simulink subsystem "ElectricalThermalSystem"  (R2025b)
settings: Solver=VariableStepAuto  StartTime=0.0  StopTime=10.0  RelTol=1e-3
undefined symbols (not defined in the file): EnvAirTemp, PlantThrEstCmpPwr, PlntThrAirBpt, PlntThrAirCond, PlntThrAirCp, PlntThrAirCpBpt, PlntThrAirPrand, PlntThrAirRho, PlntThrAirVisc, PlntThrBattDCFlwRatio, PlntThrBattJacLen, PlntThrChArea, PlntThrChDia, PlntThrCoolCond, PlntThrCoolCp, PlntThrCoolCpBpt, PlntThrCoolPrand, PlntThrCoolRho, PlntThrCoolVisc, PlntThrDCJacLen, PlntThrEMJacLen, PlntThrEstCOPLut, PlntThrEstDTLut, PlntThrHeaterMaxPwr, PlntThrPmpDisp, PlntThrPmpHeadP, PlntThrPmpMaxSpd, PlntThrPmpMechEff, PlntThrPmpVolEff, PlntThrRadAirArea, PlntThrRadAirDh, PlntThrRadFanAreaFlw, PlntThrRadFlwCoef, PlntThrRadGapHeight, PlntThrRadLength, PlntThrRadNTubes, PlntThrRadTubeDh, PlntThrRadTubeHeight, PlntThrRadWidth
libraries: autolibutils x62
(part 4 of 4)

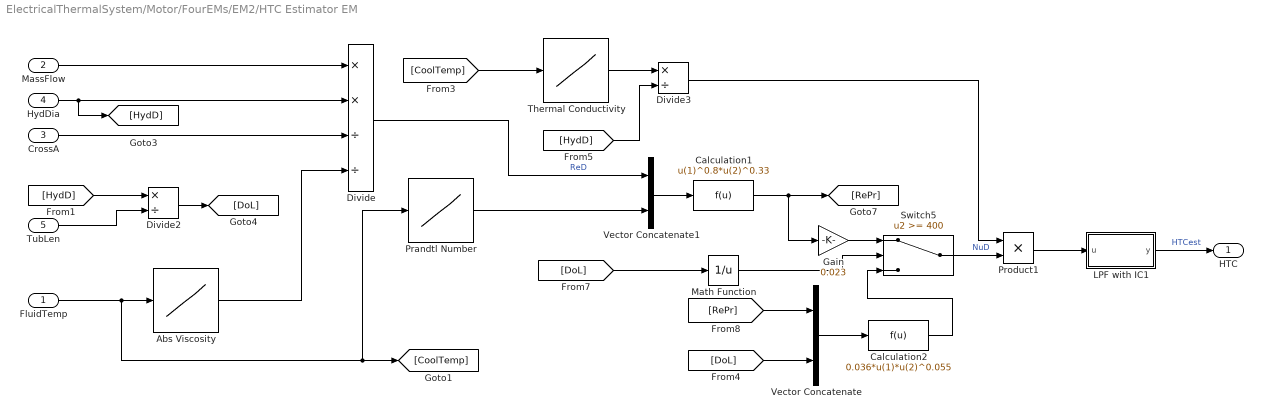
== system ElectricalThermalSystem/Motor/FourEMs/EM2/HTC Estimator EM ==
  FluidTemp : Inport
  MassFlow : Inport  Port=2
  CrossA : Inport  Port=3  OutMin=eps
  HydDia : Inport  Port=4
  TubLen : Inport  Port=5
  Abs Viscosity : Lookup_n-D  NumberOfTableDimensions=1  BreakpointsForDimension1=PlntThrCoolCpBpt  Table=PlntThrCoolVisc  ExtrapMethod=Clip  UseLastTableValue=on  InternalRulePriority=Speed  RndMeth=Simplest
  Calculation1 : Fcn  Expr=u(1)^0.8*u(2)^0.33
  Calculation2 : Fcn  Expr=0.036*u(1)*u(2)^0.055
  Divide : Product  Inputs=**//
  Divide2 : Product  Inputs=*/
  Divide3 : Product  Inputs=*/
  Gain : Gain  Gain=0.023
  LPF with IC1 : Subsystem  mask{wc=10, InitCond=10, dataType=off}
      mask prompts: wc "Cutoff frequency, wc [rad/s]"; InitCond "Initial condition, InitCond [same as u]"; dataType "Enforce same input data type"
      mask TypeOptions wc: Cont LPF IC/wc
      mask TypeOptions InitCond: Initial Condition/Value
      mask TypeOptions dataType: Cont LPF IC/dataType
  Math Function : Math  Operator=reciprocal
  Prandtl Number : Lookup_n-D  NumberOfTableDimensions=1  BreakpointsForDimension1=PlntThrCoolCpBpt  Table=PlntThrCoolPrand  ExtrapMethod=Clip  UseLastTableValue=on  InternalRulePriority=Speed  RndMeth=Simplest
  Product1 : Product
  Switch5 : Switch  Threshold=400  SaturateOnIntegerOverflow=off  InputSameDT=off
  Thermal Conductivity : Lookup_n-D  NumberOfTableDimensions=1  BreakpointsForDimension1=PlntThrCoolCpBpt  Table=PlntThrCoolCond  ExtrapMethod=Clip  UseLastTableValue=on  InternalRulePriority=Speed  RndMeth=Simplest
  Vector Concatenate : Concatenate
  Vector Concatenate1 : Concatenate
  HTC : Outport
  wires:
  LPF with IC1/1(y) -> HTC/1  "HTCest"
  FluidTemp/1 -> Prandtl Number/1, [CoolTemp], Abs Viscosity/1
  [CoolTemp] -> Thermal Conductivity/1
  MassFlow/1 -> Divide/1
  HydDia/1 -> [HydD], Divide/2
  CrossA/1 -> Divide/3
  [HydD] -> Divide2/1
  TubLen/1 -> Divide2/2
  Divide2/1 -> [DoL]
  Abs Viscosity/1 -> Divide/4
  Divide/1 -> Vector Concatenate1/1  "ReD"
  Prandtl Number/1 -> Vector Concatenate1/2
  Vector Concatenate1/1 -> Calculation1/1
  [DoL] -> Math Function/1
  Math Function/1 -> Switch5/2
  Thermal Conductivity/1 -> Divide3/1
  [HydD] -> Divide3/2
  Divide3/1 -> Product1/1
  Gain/1 -> Switch5/1
  Calculation1/1 -> [RePr], Gain/1
  [RePr] -> Vector Concatenate/1
  [DoL] -> Vector Concatenate/2
  Vector Concatenate/1 -> Calculation2/1
  Calculation2/1 -> Switch5/3
  Switch5/1 -> Product1/2  "NuD"
  Product1/1 -> LPF with IC1/1(u)

== system ElectricalThermalSystem/Motor/FourEMs/EM2/Temperature and Heat Flow ==
  HTC : Inport
  CoolTempIn : Inport  Port=2
  EMTemp : Inport  Port=3
  CoolMflw : Inport  Port=4
  JacArea : Inport  Port=5
  Divide2 : Product  Inputs=*/
  Gain4 : Gain  Gain=0.5
  LPF with IC1 : Subsystem  mask{wc=10, InitCond=EnvAirTemp, dataType=off}
      mask prompts: wc "Cutoff frequency, wc [rad/s]"; InitCond "Initial condition, InitCond [same as u]"; dataType "Enforce same input data type"
      mask TypeOptions wc: Cont LPF IC/wc
      mask TypeOptions InitCond: Initial Condition/Value
      mask TypeOptions dataType: Cont LPF IC/dataType
  Minus3 : Sum
  Minus4 : Sum
  Product1 : Product  Inputs=3
  Product2 : Product
  Selector : Selector  InputPortWidth=PlntEMNum  IndexOptions=Index vector (dialog)  Indices=2  OutputSizes=1
  Specific Heat 2 : Lookup_n-D  NumberOfTableDimensions=1  BreakpointsForDimension1=PlntThrCoolCpBpt  Table=PlntThrCoolCp  ExtrapMethod=Clip  UseLastTableValue=on  InternalRulePriority=Speed  RndMeth=Simplest
  Subtract : Sum  Inputs=+-
  div0protect - abs poly4 : autolibutils/div0protect - abs poly  thresh=.001  aMode=1
  BulkCoolTemp : Outport
  Qem : Outport  Port=2
  CoolTempOut : Outport  Port=3
  wires:
  LPF with IC1/1(y) -> BulkCoolTemp/1, [BulkCoolTemp]
  EMTemp/1 -> Selector/1
  HTC/1 -> Product1/1
  Product2/1 -> div0protect - abs poly4/1
  Minus4/1 -> Gain4/1
  Gain4/1 -> LPF with IC1/1(u)
  Minus3/1 -> Minus4/2, CoolTempOut/1
  Product1/1 -> Divide2/1, Qem/1  "Qem"
  JacArea/1 -> Product1/2
  div0protect - abs poly4/1 -> Divide2/2
  Specific Heat 2/1 -> Product2/2
  [BulkCoolTemp] -> Specific Heat 2/1, Subtract/2
  Subtract/1 -> Product1/3
  Selector/1 -> Subtract/1
  Divide2/1 -> Minus3/2
  CoolMflw/1 -> Product2/1
  CoolTempIn/1 -> Minus4/1, Minus3/1

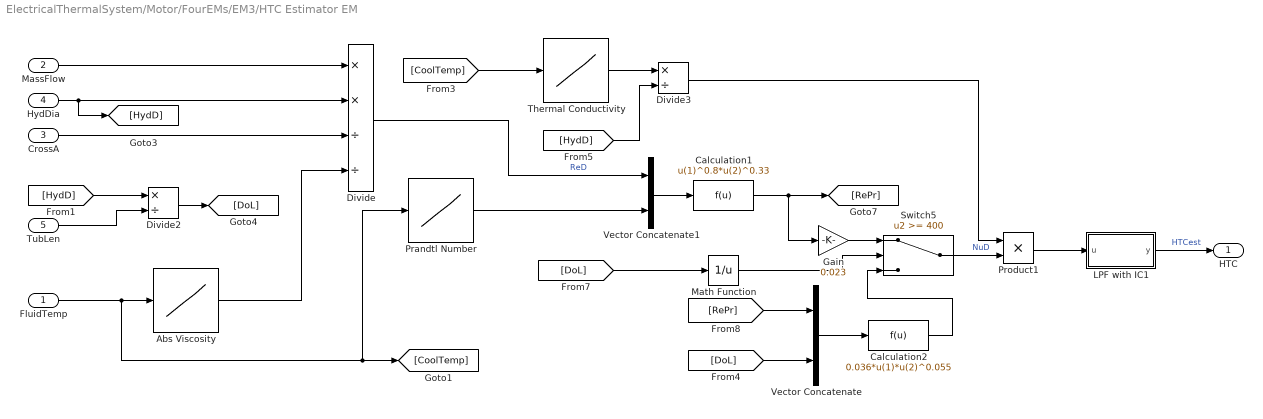
== system ElectricalThermalSystem/Motor/FourEMs/EM3/HTC Estimator EM ==
  FluidTemp : Inport
  MassFlow : Inport  Port=2
  CrossA : Inport  Port=3  OutMin=eps
  HydDia : Inport  Port=4
  TubLen : Inport  Port=5
  Abs Viscosity : Lookup_n-D  NumberOfTableDimensions=1  BreakpointsForDimension1=PlntThrCoolCpBpt  Table=PlntThrCoolVisc  ExtrapMethod=Clip  UseLastTableValue=on  InternalRulePriority=Speed  RndMeth=Simplest
  Calculation1 : Fcn  Expr=u(1)^0.8*u(2)^0.33
  Calculation2 : Fcn  Expr=0.036*u(1)*u(2)^0.055
  Divide : Product  Inputs=**//
  Divide2 : Product  Inputs=*/
  Divide3 : Product  Inputs=*/
  Gain : Gain  Gain=0.023
  LPF with IC1 : Subsystem  mask{wc=10, InitCond=10, dataType=off}
      mask prompts: wc "Cutoff frequency, wc [rad/s]"; InitCond "Initial condition, InitCond [same as u]"; dataType "Enforce same input data type"
      mask TypeOptions wc: Cont LPF IC/wc
      mask TypeOptions InitCond: Initial Condition/Value
      mask TypeOptions dataType: Cont LPF IC/dataType
  Math Function : Math  Operator=reciprocal
  Prandtl Number : Lookup_n-D  NumberOfTableDimensions=1  BreakpointsForDimension1=PlntThrCoolCpBpt  Table=PlntThrCoolPrand  ExtrapMethod=Clip  UseLastTableValue=on  InternalRulePriority=Speed  RndMeth=Simplest
  Product1 : Product
  Switch5 : Switch  Threshold=400  SaturateOnIntegerOverflow=off  InputSameDT=off
  Thermal Conductivity : Lookup_n-D  NumberOfTableDimensions=1  BreakpointsForDimension1=PlntThrCoolCpBpt  Table=PlntThrCoolCond  ExtrapMethod=Clip  UseLastTableValue=on  InternalRulePriority=Speed  RndMeth=Simplest
  Vector Concatenate : Concatenate
  Vector Concatenate1 : Concatenate
  HTC : Outport
  wires:
  LPF with IC1/1(y) -> HTC/1  "HTCest"
  FluidTemp/1 -> Prandtl Number/1, [CoolTemp], Abs Viscosity/1
  [CoolTemp] -> Thermal Conductivity/1
  MassFlow/1 -> Divide/1
  HydDia/1 -> [HydD], Divide/2
  CrossA/1 -> Divide/3
  [HydD] -> Divide2/1
  TubLen/1 -> Divide2/2
  Divide2/1 -> [DoL]
  Abs Viscosity/1 -> Divide/4
  Divide/1 -> Vector Concatenate1/1  "ReD"
  Prandtl Number/1 -> Vector Concatenate1/2
  Vector Concatenate1/1 -> Calculation1/1
  [DoL] -> Math Function/1
  Math Function/1 -> Switch5/2
  Thermal Conductivity/1 -> Divide3/1
  [HydD] -> Divide3/2
  Divide3/1 -> Product1/1
  Gain/1 -> Switch5/1
  Calculation1/1 -> [RePr], Gain/1
  [RePr] -> Vector Concatenate/1
  [DoL] -> Vector Concatenate/2
  Vector Concatenate/1 -> Calculation2/1
  Calculation2/1 -> Switch5/3
  Switch5/1 -> Product1/2  "NuD"
  Product1/1 -> LPF with IC1/1(u)

== system ElectricalThermalSystem/Motor/FourEMs/EM3/Temperature and Heat Flow ==
  HTC : Inport
  CoolTempIn : Inport  Port=2
  EMTemp : Inport  Port=3
  CoolMflw : Inport  Port=4
  JacArea : Inport  Port=5
  Divide2 : Product  Inputs=*/
  Gain4 : Gain  Gain=0.5
  LPF with IC1 : Subsystem  mask{wc=10, InitCond=EnvAirTemp, dataType=off}
      mask prompts: wc "Cutoff frequency, wc [rad/s]"; InitCond "Initial condition, InitCond [same as u]"; dataType "Enforce same input data type"
      mask TypeOptions wc: Cont LPF IC/wc
      mask TypeOptions InitCond: Initial Condition/Value
      mask TypeOptions dataType: Cont LPF IC/dataType
  Minus3 : Sum
  Minus4 : Sum
  Product1 : Product  Inputs=3
  Product2 : Product
  Selector : Selector  InputPortWidth=PlntEMNum  IndexOptions=Index vector (dialog)  Indices=3  OutputSizes=1
  Specific Heat 2 : Lookup_n-D  NumberOfTableDimensions=1  BreakpointsForDimension1=PlntThrCoolCpBpt  Table=PlntThrCoolCp  ExtrapMethod=Clip  UseLastTableValue=on  InternalRulePriority=Speed  RndMeth=Simplest
  Subtract : Sum  Inputs=+-
  div0protect - abs poly4 : autolibutils/div0protect - abs poly  thresh=.001  aMode=1
  BulkCoolTemp : Outport
  Qem : Outport  Port=2
  CoolTempOut : Outport  Port=3
  wires:
  LPF with IC1/1(y) -> BulkCoolTemp/1, [BulkCoolTemp]
  EMTemp/1 -> Selector/1
  HTC/1 -> Product1/1
  Product2/1 -> div0protect - abs poly4/1
  Minus4/1 -> Gain4/1
  Gain4/1 -> LPF with IC1/1(u)
  Minus3/1 -> Minus4/2, CoolTempOut/1
  Product1/1 -> Divide2/1, Qem/1  "Qem"
  JacArea/1 -> Product1/2
  div0protect - abs poly4/1 -> Divide2/2
  Specific Heat 2/1 -> Product2/2
  [BulkCoolTemp] -> Specific Heat 2/1, Subtract/2
  Subtract/1 -> Product1/3
  Selector/1 -> Subtract/1
  Divide2/1 -> Minus3/2
  CoolMflw/1 -> Product2/1
  CoolTempIn/1 -> Minus4/1, Minus3/1

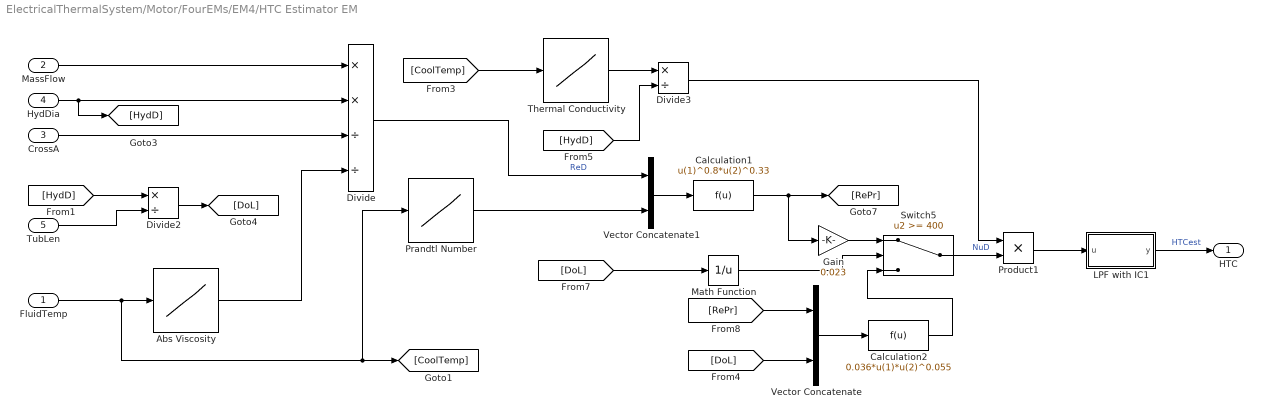
== system ElectricalThermalSystem/Motor/FourEMs/EM4/HTC Estimator EM ==
  FluidTemp : Inport
  MassFlow : Inport  Port=2
  CrossA : Inport  Port=3  OutMin=eps
  HydDia : Inport  Port=4
  TubLen : Inport  Port=5
  Abs Viscosity : Lookup_n-D  NumberOfTableDimensions=1  BreakpointsForDimension1=PlntThrCoolCpBpt  Table=PlntThrCoolVisc  ExtrapMethod=Clip  UseLastTableValue=on  InternalRulePriority=Speed  RndMeth=Simplest
  Calculation1 : Fcn  Expr=u(1)^0.8*u(2)^0.33
  Calculation2 : Fcn  Expr=0.036*u(1)*u(2)^0.055
  Divide : Product  Inputs=**//
  Divide2 : Product  Inputs=*/
  Divide3 : Product  Inputs=*/
  Gain : Gain  Gain=0.023
  LPF with IC1 : Subsystem  mask{wc=10, InitCond=10, dataType=off}
      mask prompts: wc "Cutoff frequency, wc [rad/s]"; InitCond "Initial condition, InitCond [same as u]"; dataType "Enforce same input data type"
      mask TypeOptions wc: Cont LPF IC/wc
      mask TypeOptions InitCond: Initial Condition/Value
      mask TypeOptions dataType: Cont LPF IC/dataType
  Math Function : Math  Operator=reciprocal
  Prandtl Number : Lookup_n-D  NumberOfTableDimensions=1  BreakpointsForDimension1=PlntThrCoolCpBpt  Table=PlntThrCoolPrand  ExtrapMethod=Clip  UseLastTableValue=on  InternalRulePriority=Speed  RndMeth=Simplest
  Product1 : Product
  Switch5 : Switch  Threshold=400  SaturateOnIntegerOverflow=off  InputSameDT=off
  Thermal Conductivity : Lookup_n-D  NumberOfTableDimensions=1  BreakpointsForDimension1=PlntThrCoolCpBpt  Table=PlntThrCoolCond  ExtrapMethod=Clip  UseLastTableValue=on  InternalRulePriority=Speed  RndMeth=Simplest
  Vector Concatenate : Concatenate
  Vector Concatenate1 : Concatenate
  HTC : Outport
  wires:
  LPF with IC1/1(y) -> HTC/1  "HTCest"
  FluidTemp/1 -> Prandtl Number/1, [CoolTemp], Abs Viscosity/1
  [CoolTemp] -> Thermal Conductivity/1
  MassFlow/1 -> Divide/1
  HydDia/1 -> [HydD], Divide/2
  CrossA/1 -> Divide/3
  [HydD] -> Divide2/1
  TubLen/1 -> Divide2/2
  Divide2/1 -> [DoL]
  Abs Viscosity/1 -> Divide/4
  Divide/1 -> Vector Concatenate1/1  "ReD"
  Prandtl Number/1 -> Vector Concatenate1/2
  Vector Concatenate1/1 -> Calculation1/1
  [DoL] -> Math Function/1
  Math Function/1 -> Switch5/2
  Thermal Conductivity/1 -> Divide3/1
  [HydD] -> Divide3/2
  Divide3/1 -> Product1/1
  Gain/1 -> Switch5/1
  Calculation1/1 -> [RePr], Gain/1
  [RePr] -> Vector Concatenate/1
  [DoL] -> Vector Concatenate/2
  Vector Concatenate/1 -> Calculation2/1
  Calculation2/1 -> Switch5/3
  Switch5/1 -> Product1/2  "NuD"
  Product1/1 -> LPF with IC1/1(u)

== system ElectricalThermalSystem/Motor/FourEMs/EM4/Temperature and Heat Flow ==
  HTC : Inport
  CoolTempIn : Inport  Port=2
  EMTemp : Inport  Port=3
  CoolMflw : Inport  Port=4
  JacArea : Inport  Port=5
  Divide2 : Product  Inputs=*/
  Gain4 : Gain  Gain=0.5
  LPF with IC1 : Subsystem  mask{wc=10, InitCond=EnvAirTemp, dataType=off}
      mask prompts: wc "Cutoff frequency, wc [rad/s]"; InitCond "Initial condition, InitCond [same as u]"; dataType "Enforce same input data type"
      mask TypeOptions wc: Cont LPF IC/wc
      mask TypeOptions InitCond: Initial Condition/Value
      mask TypeOptions dataType: Cont LPF IC/dataType
  Minus3 : Sum
  Minus4 : Sum
  Product1 : Product  Inputs=3
  Product2 : Product
  Selector : Selector  InputPortWidth=PlntEMNum  IndexOptions=Index vector (dialog)  Indices=4  OutputSizes=1
  Specific Heat 2 : Lookup_n-D  NumberOfTableDimensions=1  BreakpointsForDimension1=PlntThrCoolCpBpt  Table=PlntThrCoolCp  ExtrapMethod=Clip  UseLastTableValue=on  InternalRulePriority=Speed  RndMeth=Simplest
  Subtract : Sum  Inputs=+-
  div0protect - abs poly4 : autolibutils/div0protect - abs poly  thresh=.001  aMode=1
  BulkCoolTemp : Outport
  Qem : Outport  Port=2
  CoolTempOut : Outport  Port=3
  wires:
  LPF with IC1/1(y) -> BulkCoolTemp/1, [BulkCoolTemp]
  EMTemp/1 -> Selector/1
  HTC/1 -> Product1/1
  Product2/1 -> div0protect - abs poly4/1
  Minus4/1 -> Gain4/1
  Gain4/1 -> LPF with IC1/1(u)
  Minus3/1 -> Minus4/2, CoolTempOut/1
  Product1/1 -> Divide2/1, Qem/1  "Qem"
  JacArea/1 -> Product1/2
  div0protect - abs poly4/1 -> Divide2/2
  Specific Heat 2/1 -> Product2/2
  [BulkCoolTemp] -> Specific Heat 2/1, Subtract/2
  Subtract/1 -> Product1/3
  Selector/1 -> Subtract/1
  Divide2/1 -> Minus3/2
  CoolMflw/1 -> Product2/1
  CoolTempIn/1 -> Minus4/1, Minus3/1

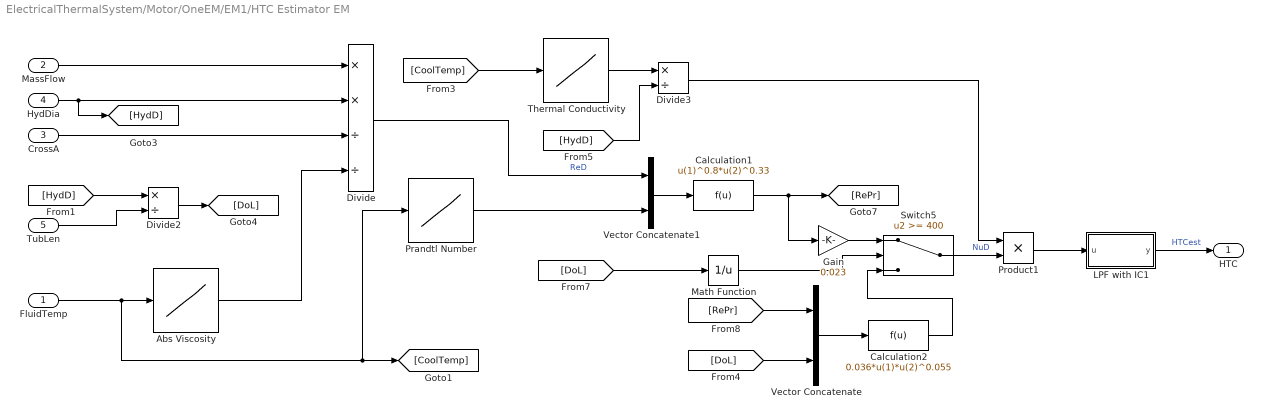
== system ElectricalThermalSystem/Motor/OneEM/EM1/HTC Estimator EM ==
  FluidTemp : Inport
  MassFlow : Inport  Port=2
  CrossA : Inport  Port=3  OutMin=eps
  HydDia : Inport  Port=4
  TubLen : Inport  Port=5
  Abs Viscosity : Lookup_n-D  NumberOfTableDimensions=1  BreakpointsForDimension1=PlntThrCoolCpBpt  Table=PlntThrCoolVisc  ExtrapMethod=Clip  UseLastTableValue=on  InternalRulePriority=Speed  RndMeth=Simplest
  Calculation1 : Fcn  Expr=u(1)^0.8*u(2)^0.33
  Calculation2 : Fcn  Expr=0.036*u(1)*u(2)^0.055
  Divide : Product  Inputs=**//
  Divide2 : Product  Inputs=*/
  Divide3 : Product  Inputs=*/
  Gain : Gain  Gain=0.023
  LPF with IC1 : Subsystem  mask{wc=10, InitCond=10, dataType=off}
      mask prompts: wc "Cutoff frequency, wc [rad/s]"; InitCond "Initial condition, InitCond [same as u]"; dataType "Enforce same input data type"
      mask TypeOptions wc: Cont LPF IC/wc
      mask TypeOptions InitCond: Initial Condition/Value
      mask TypeOptions dataType: Cont LPF IC/dataType
  Math Function : Math  Operator=reciprocal
  Prandtl Number : Lookup_n-D  NumberOfTableDimensions=1  BreakpointsForDimension1=PlntThrCoolCpBpt  Table=PlntThrCoolPrand  ExtrapMethod=Clip  UseLastTableValue=on  InternalRulePriority=Speed  RndMeth=Simplest
  Product1 : Product
  Switch5 : Switch  Threshold=400  SaturateOnIntegerOverflow=off  InputSameDT=off
  Thermal Conductivity : Lookup_n-D  NumberOfTableDimensions=1  BreakpointsForDimension1=PlntThrCoolCpBpt  Table=PlntThrCoolCond  ExtrapMethod=Clip  UseLastTableValue=on  InternalRulePriority=Speed  RndMeth=Simplest
  Vector Concatenate : Concatenate
  Vector Concatenate1 : Concatenate
  HTC : Outport
  wires:
  LPF with IC1/1(y) -> HTC/1  "HTCest"
  FluidTemp/1 -> Prandtl Number/1, [CoolTemp], Abs Viscosity/1
  [CoolTemp] -> Thermal Conductivity/1
  MassFlow/1 -> Divide/1
  HydDia/1 -> [HydD], Divide/2
  CrossA/1 -> Divide/3
  [HydD] -> Divide2/1
  TubLen/1 -> Divide2/2
  Divide2/1 -> [DoL]
  Abs Viscosity/1 -> Divide/4
  Divide/1 -> Vector Concatenate1/1  "ReD"
  Prandtl Number/1 -> Vector Concatenate1/2
  Vector Concatenate1/1 -> Calculation1/1
  [DoL] -> Math Function/1
  Math Function/1 -> Switch5/2
  Thermal Conductivity/1 -> Divide3/1
  [HydD] -> Divide3/2
  Divide3/1 -> Product1/1
  Gain/1 -> Switch5/1
  Calculation1/1 -> [RePr], Gain/1
  [RePr] -> Vector Concatenate/1
  [DoL] -> Vector Concatenate/2
  Vector Concatenate/1 -> Calculation2/1
  Calculation2/1 -> Switch5/3
  Switch5/1 -> Product1/2  "NuD"
  Product1/1 -> LPF with IC1/1(u)

== system ElectricalThermalSystem/Motor/OneEM/EM1/Temperature and Heat Flow ==
  HTC : Inport
  CoolTempIn : Inport  Port=2
  EMTemp : Inport  Port=3
  CoolMflw : Inport  Port=4
  JacArea : Inport  Port=5
  Divide2 : Product  Inputs=*/
  Gain4 : Gain  Gain=0.5
  LPF with IC1 : Subsystem  mask{wc=10, InitCond=EnvAirTemp, dataType=off}
      mask prompts: wc "Cutoff frequency, wc [rad/s]"; InitCond "Initial condition, InitCond [same as u]"; dataType "Enforce same input data type"
      mask TypeOptions wc: Cont LPF IC/wc
      mask TypeOptions InitCond: Initial Condition/Value
      mask TypeOptions dataType: Cont LPF IC/dataType
  Minus3 : Sum
  Minus4 : Sum
  Product1 : Product  Inputs=3
  Product2 : Product
  Selector : Selector  InputPortWidth=PlntEMNum  IndexOptions=Index vector (dialog)  Indices=1  OutputSizes=1
  Specific Heat 2 : Lookup_n-D  NumberOfTableDimensions=1  BreakpointsForDimension1=PlntThrCoolCpBpt  Table=PlntThrCoolCp  ExtrapMethod=Clip  UseLastTableValue=on  InternalRulePriority=Speed  RndMeth=Simplest
  Subtract : Sum  Inputs=+-
  div0protect - abs poly4 : autolibutils/div0protect - abs poly  thresh=.001  aMode=1
  BulkCoolTemp : Outport
  Qem : Outport  Port=2
  CoolTempOut : Outport  Port=3
  wires:
  LPF with IC1/1(y) -> BulkCoolTemp/1, [BulkCoolTemp]
  EMTemp/1 -> Selector/1
  HTC/1 -> Product1/1
  Product2/1 -> div0protect - abs poly4/1
  Minus4/1 -> Gain4/1
  Gain4/1 -> LPF with IC1/1(u)
  Minus3/1 -> Minus4/2, CoolTempOut/1
  Product1/1 -> Divide2/1, Qem/1  "Qem"
  JacArea/1 -> Product1/2
  div0protect - abs poly4/1 -> Divide2/2
  Specific Heat 2/1 -> Product2/2
  [BulkCoolTemp] -> Specific Heat 2/1, Subtract/2
  Subtract/1 -> Product1/3
  Selector/1 -> Subtract/1
  Divide2/1 -> Minus3/2
  CoolMflw/1 -> Product2/1
  CoolTempIn/1 -> Minus4/1, Minus3/1

== system ElectricalThermalSystem/Motor/ThreeEMs/EM1/HTC Estimator EM ==
  FluidTemp : Inport
  MassFlow : Inport  Port=2
  CrossA : Inport  Port=3  OutMin=eps
  HydDia : Inport  Port=4
  TubLen : Inport  Port=5
  Abs Viscosity : Lookup_n-D  NumberOfTableDimensions=1  BreakpointsForDimension1=PlntThrCoolCpBpt  Table=PlntThrCoolVisc  ExtrapMethod=Clip  UseLastTableValue=on  InternalRulePriority=Speed  RndMeth=Simplest
  Calculation1 : Fcn  Expr=u(1)^0.8*u(2)^0.33
  Calculation2 : Fcn  Expr=0.036*u(1)*u(2)^0.055
  Divide : Product  Inputs=**//
  Divide2 : Product  Inputs=*/
  Divide3 : Product  Inputs=*/
  Gain : Gain  Gain=0.023
  LPF with IC1 : Subsystem  mask{wc=10, InitCond=10, dataType=off}
      mask prompts: wc "Cutoff frequency, wc [rad/s]"; InitCond "Initial condition, InitCond [same as u]"; dataType "Enforce same input data type"
      mask TypeOptions wc: Cont LPF IC/wc
      mask TypeOptions InitCond: Initial Condition/Value
      mask TypeOptions dataType: Cont LPF IC/dataType
  Math Function : Math  Operator=reciprocal
  Prandtl Number : Lookup_n-D  NumberOfTableDimensions=1  BreakpointsForDimension1=PlntThrCoolCpBpt  Table=PlntThrCoolPrand  ExtrapMethod=Clip  UseLastTableValue=on  InternalRulePriority=Speed  RndMeth=Simplest
  Product1 : Product
  Switch5 : Switch  Threshold=400  SaturateOnIntegerOverflow=off  InputSameDT=off
  Thermal Conductivity : Lookup_n-D  NumberOfTableDimensions=1  BreakpointsForDimension1=PlntThrCoolCpBpt  Table=PlntThrCoolCond  ExtrapMethod=Clip  UseLastTableValue=on  InternalRulePriority=Speed  RndMeth=Simplest
  Vector Concatenate : Concatenate
  Vector Concatenate1 : Concatenate
  HTC : Outport
  wires:
  LPF with IC1/1(y) -> HTC/1  "HTCest"
  FluidTemp/1 -> Prandtl Number/1, [CoolTemp], Abs Viscosity/1
  [CoolTemp] -> Thermal Conductivity/1
  MassFlow/1 -> Divide/1
  HydDia/1 -> [HydD], Divide/2
  CrossA/1 -> Divide/3
  [HydD] -> Divide2/1
  TubLen/1 -> Divide2/2
  Divide2/1 -> [DoL]
  Abs Viscosity/1 -> Divide/4
  Divide/1 -> Vector Concatenate1/1  "ReD"
  Prandtl Number/1 -> Vector Concatenate1/2
  Vector Concatenate1/1 -> Calculation1/1
  [DoL] -> Math Function/1
  Math Function/1 -> Switch5/2
  Thermal Conductivity/1 -> Divide3/1
  [HydD] -> Divide3/2
  Divide3/1 -> Product1/1
  Gain/1 -> Switch5/1
  Calculation1/1 -> [RePr], Gain/1
  [RePr] -> Vector Concatenate/1
  [DoL] -> Vector Concatenate/2
  Vector Concatenate/1 -> Calculation2/1
  Calculation2/1 -> Switch5/3
  Switch5/1 -> Product1/2  "NuD"
  Product1/1 -> LPF with IC1/1(u)

== system ElectricalThermalSystem/Motor/ThreeEMs/EM1/Temperature and Heat Flow ==
  HTC : Inport
  CoolTempIn : Inport  Port=2
  EMTemp : Inport  Port=3
  CoolMflw : Inport  Port=4
  JacArea : Inport  Port=5
  Divide2 : Product  Inputs=*/
  Gain4 : Gain  Gain=0.5
  LPF with IC1 : Subsystem  mask{wc=10, InitCond=EnvAirTemp, dataType=off}
      mask prompts: wc "Cutoff frequency, wc [rad/s]"; InitCond "Initial condition, InitCond [same as u]"; dataType "Enforce same input data type"
      mask TypeOptions wc: Cont LPF IC/wc
      mask TypeOptions InitCond: Initial Condition/Value
      mask TypeOptions dataType: Cont LPF IC/dataType
  Minus3 : Sum
  Minus4 : Sum
  Product1 : Product  Inputs=3
  Product2 : Product
  Selector : Selector  InputPortWidth=PlntEMNum  IndexOptions=Index vector (dialog)  Indices=1  OutputSizes=1
  Specific Heat 2 : Lookup_n-D  NumberOfTableDimensions=1  BreakpointsForDimension1=PlntThrCoolCpBpt  Table=PlntThrCoolCp  ExtrapMethod=Clip  UseLastTableValue=on  InternalRulePriority=Speed  RndMeth=Simplest
  Subtract : Sum  Inputs=+-
  div0protect - abs poly4 : autolibutils/div0protect - abs poly  thresh=.001  aMode=1
  BulkCoolTemp : Outport
  Qem : Outport  Port=2
  CoolTempOut : Outport  Port=3
  wires:
  LPF with IC1/1(y) -> BulkCoolTemp/1, [BulkCoolTemp]
  EMTemp/1 -> Selector/1
  HTC/1 -> Product1/1
  Product2/1 -> div0protect - abs poly4/1
  Minus4/1 -> Gain4/1
  Gain4/1 -> LPF with IC1/1(u)
  Minus3/1 -> Minus4/2, CoolTempOut/1
  Product1/1 -> Divide2/1, Qem/1  "Qem"
  JacArea/1 -> Product1/2
  div0protect - abs poly4/1 -> Divide2/2
  Specific Heat 2/1 -> Product2/2
  [BulkCoolTemp] -> Specific Heat 2/1, Subtract/2
  Subtract/1 -> Product1/3
  Selector/1 -> Subtract/1
  Divide2/1 -> Minus3/2
  CoolMflw/1 -> Product2/1
  CoolTempIn/1 -> Minus4/1, Minus3/1

== system ElectricalThermalSystem/Motor/ThreeEMs/EM2/HTC Estimator EM ==
  FluidTemp : Inport
  MassFlow : Inport  Port=2
  CrossA : Inport  Port=3  OutMin=eps
  HydDia : Inport  Port=4
  TubLen : Inport  Port=5
  Abs Viscosity : Lookup_n-D  NumberOfTableDimensions=1  BreakpointsForDimension1=PlntThrCoolCpBpt  Table=PlntThrCoolVisc  ExtrapMethod=Clip  UseLastTableValue=on  InternalRulePriority=Speed  RndMeth=Simplest
  Calculation1 : Fcn  Expr=u(1)^0.8*u(2)^0.33
  Calculation2 : Fcn  Expr=0.036*u(1)*u(2)^0.055
  Divide : Product  Inputs=**//
  Divide2 : Product  Inputs=*/
  Divide3 : Product  Inputs=*/
  Gain : Gain  Gain=0.023
  LPF with IC1 : Subsystem  mask{wc=10, InitCond=10, dataType=off}
      mask prompts: wc "Cutoff frequency, wc [rad/s]"; InitCond "Initial condition, InitCond [same as u]"; dataType "Enforce same input data type"
      mask TypeOptions wc: Cont LPF IC/wc
      mask TypeOptions InitCond: Initial Condition/Value
      mask TypeOptions dataType: Cont LPF IC/dataType
  Math Function : Math  Operator=reciprocal
  Prandtl Number : Lookup_n-D  NumberOfTableDimensions=1  BreakpointsForDimension1=PlntThrCoolCpBpt  Table=PlntThrCoolPrand  ExtrapMethod=Clip  UseLastTableValue=on  InternalRulePriority=Speed  RndMeth=Simplest
  Product1 : Product
  Switch5 : Switch  Threshold=400  SaturateOnIntegerOverflow=off  InputSameDT=off
  Thermal Conductivity : Lookup_n-D  NumberOfTableDimensions=1  BreakpointsForDimension1=PlntThrCoolCpBpt  Table=PlntThrCoolCond  ExtrapMethod=Clip  UseLastTableValue=on  InternalRulePriority=Speed  RndMeth=Simplest
  Vector Concatenate : Concatenate
  Vector Concatenate1 : Concatenate
  HTC : Outport
  wires:
  LPF with IC1/1(y) -> HTC/1  "HTCest"
  FluidTemp/1 -> Prandtl Number/1, [CoolTemp], Abs Viscosity/1
  [CoolTemp] -> Thermal Conductivity/1
  MassFlow/1 -> Divide/1
  HydDia/1 -> [HydD], Divide/2
  CrossA/1 -> Divide/3
  [HydD] -> Divide2/1
  TubLen/1 -> Divide2/2
  Divide2/1 -> [DoL]
  Abs Viscosity/1 -> Divide/4
  Divide/1 -> Vector Concatenate1/1  "ReD"
  Prandtl Number/1 -> Vector Concatenate1/2
  Vector Concatenate1/1 -> Calculation1/1
  [DoL] -> Math Function/1
  Math Function/1 -> Switch5/2
  Thermal Conductivity/1 -> Divide3/1
  [HydD] -> Divide3/2
  Divide3/1 -> Product1/1
  Gain/1 -> Switch5/1
  Calculation1/1 -> [RePr], Gain/1
  [RePr] -> Vector Concatenate/1
  [DoL] -> Vector Concatenate/2
  Vector Concatenate/1 -> Calculation2/1
  Calculation2/1 -> Switch5/3
  Switch5/1 -> Product1/2  "NuD"
  Product1/1 -> LPF with IC1/1(u)

== system ElectricalThermalSystem/Motor/ThreeEMs/EM2/Temperature and Heat Flow ==
  HTC : Inport
  CoolTempIn : Inport  Port=2
  EMTemp : Inport  Port=3
  CoolMflw : Inport  Port=4
  JacArea : Inport  Port=5
  Divide2 : Product  Inputs=*/
  Gain4 : Gain  Gain=0.5
  LPF with IC1 : Subsystem  mask{wc=10, InitCond=EnvAirTemp, dataType=off}
      mask prompts: wc "Cutoff frequency, wc [rad/s]"; InitCond "Initial condition, InitCond [same as u]"; dataType "Enforce same input data type"
      mask TypeOptions wc: Cont LPF IC/wc
      mask TypeOptions InitCond: Initial Condition/Value
      mask TypeOptions dataType: Cont LPF IC/dataType
  Minus3 : Sum
  Minus4 : Sum
  Product1 : Product  Inputs=3
  Product2 : Product
  Selector : Selector  InputPortWidth=PlntEMNum  IndexOptions=Index vector (dialog)  Indices=2  OutputSizes=1
  Specific Heat 2 : Lookup_n-D  NumberOfTableDimensions=1  BreakpointsForDimension1=PlntThrCoolCpBpt  Table=PlntThrCoolCp  ExtrapMethod=Clip  UseLastTableValue=on  InternalRulePriority=Speed  RndMeth=Simplest
  Subtract : Sum  Inputs=+-
  div0protect - abs poly4 : autolibutils/div0protect - abs poly  thresh=.001  aMode=1
  BulkCoolTemp : Outport
  Qem : Outport  Port=2
  CoolTempOut : Outport  Port=3
  wires:
  LPF with IC1/1(y) -> BulkCoolTemp/1, [BulkCoolTemp]
  EMTemp/1 -> Selector/1
  HTC/1 -> Product1/1
  Product2/1 -> div0protect - abs poly4/1
  Minus4/1 -> Gain4/1
  Gain4/1 -> LPF with IC1/1(u)
  Minus3/1 -> Minus4/2, CoolTempOut/1
  Product1/1 -> Divide2/1, Qem/1  "Qem"
  JacArea/1 -> Product1/2
  div0protect - abs poly4/1 -> Divide2/2
  Specific Heat 2/1 -> Product2/2
  [BulkCoolTemp] -> Specific Heat 2/1, Subtract/2
  Subtract/1 -> Product1/3
  Selector/1 -> Subtract/1
  Divide2/1 -> Minus3/2
  CoolMflw/1 -> Product2/1
  CoolTempIn/1 -> Minus4/1, Minus3/1

== system ElectricalThermalSystem/Motor/ThreeEMs/EM3/HTC Estimator EM ==
  FluidTemp : Inport
  MassFlow : Inport  Port=2
  CrossA : Inport  Port=3  OutMin=eps
  HydDia : Inport  Port=4
  TubLen : Inport  Port=5
  Abs Viscosity : Lookup_n-D  NumberOfTableDimensions=1  BreakpointsForDimension1=PlntThrCoolCpBpt  Table=PlntThrCoolVisc  ExtrapMethod=Clip  UseLastTableValue=on  InternalRulePriority=Speed  RndMeth=Simplest
  Calculation1 : Fcn  Expr=u(1)^0.8*u(2)^0.33
  Calculation2 : Fcn  Expr=0.036*u(1)*u(2)^0.055
  Divide : Product  Inputs=**//
  Divide2 : Product  Inputs=*/
  Divide3 : Product  Inputs=*/
  Gain : Gain  Gain=0.023
  LPF with IC1 : Subsystem  mask{wc=10, InitCond=10, dataType=off}
      mask prompts: wc "Cutoff frequency, wc [rad/s]"; InitCond "Initial condition, InitCond [same as u]"; dataType "Enforce same input data type"
      mask TypeOptions wc: Cont LPF IC/wc
      mask TypeOptions InitCond: Initial Condition/Value
      mask TypeOptions dataType: Cont LPF IC/dataType
  Math Function : Math  Operator=reciprocal
  Prandtl Number : Lookup_n-D  NumberOfTableDimensions=1  BreakpointsForDimension1=PlntThrCoolCpBpt  Table=PlntThrCoolPrand  ExtrapMethod=Clip  UseLastTableValue=on  InternalRulePriority=Speed  RndMeth=Simplest
  Product1 : Product
  Switch5 : Switch  Threshold=400  SaturateOnIntegerOverflow=off  InputSameDT=off
  Thermal Conductivity : Lookup_n-D  NumberOfTableDimensions=1  BreakpointsForDimension1=PlntThrCoolCpBpt  Table=PlntThrCoolCond  ExtrapMethod=Clip  UseLastTableValue=on  InternalRulePriority=Speed  RndMeth=Simplest
  Vector Concatenate : Concatenate
  Vector Concatenate1 : Concatenate
  HTC : Outport
  wires:
  LPF with IC1/1(y) -> HTC/1  "HTCest"
  FluidTemp/1 -> Prandtl Number/1, [CoolTemp], Abs Viscosity/1
  [CoolTemp] -> Thermal Conductivity/1
  MassFlow/1 -> Divide/1
  HydDia/1 -> [HydD], Divide/2
  CrossA/1 -> Divide/3
  [HydD] -> Divide2/1
  TubLen/1 -> Divide2/2
  Divide2/1 -> [DoL]
  Abs Viscosity/1 -> Divide/4
  Divide/1 -> Vector Concatenate1/1  "ReD"
  Prandtl Number/1 -> Vector Concatenate1/2
  Vector Concatenate1/1 -> Calculation1/1
  [DoL] -> Math Function/1
  Math Function/1 -> Switch5/2
  Thermal Conductivity/1 -> Divide3/1
  [HydD] -> Divide3/2
  Divide3/1 -> Product1/1
  Gain/1 -> Switch5/1
  Calculation1/1 -> [RePr], Gain/1
  [RePr] -> Vector Concatenate/1
  [DoL] -> Vector Concatenate/2
  Vector Concatenate/1 -> Calculation2/1
  Calculation2/1 -> Switch5/3
  Switch5/1 -> Product1/2  "NuD"
  Product1/1 -> LPF with IC1/1(u)

== system ElectricalThermalSystem/Motor/ThreeEMs/EM3/Temperature and Heat Flow ==
  HTC : Inport
  CoolTempIn : Inport  Port=2
  EMTemp : Inport  Port=3
  CoolMflw : Inport  Port=4
  JacArea : Inport  Port=5
  Divide2 : Product  Inputs=*/
  Gain4 : Gain  Gain=0.5
  LPF with IC1 : Subsystem  mask{wc=10, InitCond=EnvAirTemp, dataType=off}
      mask prompts: wc "Cutoff frequency, wc [rad/s]"; InitCond "Initial condition, InitCond [same as u]"; dataType "Enforce same input data type"
      mask TypeOptions wc: Cont LPF IC/wc
      mask TypeOptions InitCond: Initial Condition/Value
      mask TypeOptions dataType: Cont LPF IC/dataType
  Minus3 : Sum
  Minus4 : Sum
  Product1 : Product  Inputs=3
  Product2 : Product
  Selector : Selector  InputPortWidth=PlntEMNum  IndexOptions=Index vector (dialog)  Indices=3  OutputSizes=1
  Specific Heat 2 : Lookup_n-D  NumberOfTableDimensions=1  BreakpointsForDimension1=PlntThrCoolCpBpt  Table=PlntThrCoolCp  ExtrapMethod=Clip  UseLastTableValue=on  InternalRulePriority=Speed  RndMeth=Simplest
  Subtract : Sum  Inputs=+-
  div0protect - abs poly4 : autolibutils/div0protect - abs poly  thresh=.001  aMode=1
  BulkCoolTemp : Outport
  Qem : Outport  Port=2
  CoolTempOut : Outport  Port=3
  wires:
  LPF with IC1/1(y) -> BulkCoolTemp/1, [BulkCoolTemp]
  EMTemp/1 -> Selector/1
  HTC/1 -> Product1/1
  Product2/1 -> div0protect - abs poly4/1
  Minus4/1 -> Gain4/1
  Gain4/1 -> LPF with IC1/1(u)
  Minus3/1 -> Minus4/2, CoolTempOut/1
  Product1/1 -> Divide2/1, Qem/1  "Qem"
  JacArea/1 -> Product1/2
  div0protect - abs poly4/1 -> Divide2/2
  Specific Heat 2/1 -> Product2/2
  [BulkCoolTemp] -> Specific Heat 2/1, Subtract/2
  Subtract/1 -> Product1/3
  Selector/1 -> Subtract/1
  Divide2/1 -> Minus3/2
  CoolMflw/1 -> Product2/1
  CoolTempIn/1 -> Minus4/1, Minus3/1

== system ElectricalThermalSystem/Motor/TwoEMs/EM1/HTC Estimator EM ==
  FluidTemp : Inport
  MassFlow : Inport  Port=2
  CrossA : Inport  Port=3  OutMin=eps
  HydDia : Inport  Port=4
  TubLen : Inport  Port=5
  Abs Viscosity : Lookup_n-D  NumberOfTableDimensions=1  BreakpointsForDimension1=PlntThrCoolCpBpt  Table=PlntThrCoolVisc  ExtrapMethod=Clip  UseLastTableValue=on  InternalRulePriority=Speed  RndMeth=Simplest
  Calculation1 : Fcn  Expr=u(1)^0.8*u(2)^0.33
  Calculation2 : Fcn  Expr=0.036*u(1)*u(2)^0.055
  Divide : Product  Inputs=**//
  Divide2 : Product  Inputs=*/
  Divide3 : Product  Inputs=*/
  Gain : Gain  Gain=0.023
  LPF with IC1 : Subsystem  mask{wc=10, InitCond=10, dataType=off}
      mask prompts: wc "Cutoff frequency, wc [rad/s]"; InitCond "Initial condition, InitCond [same as u]"; dataType "Enforce same input data type"
      mask TypeOptions wc: Cont LPF IC/wc
      mask TypeOptions InitCond: Initial Condition/Value
      mask TypeOptions dataType: Cont LPF IC/dataType
  Math Function : Math  Operator=reciprocal
  Prandtl Number : Lookup_n-D  NumberOfTableDimensions=1  BreakpointsForDimension1=PlntThrCoolCpBpt  Table=PlntThrCoolPrand  ExtrapMethod=Clip  UseLastTableValue=on  InternalRulePriority=Speed  RndMeth=Simplest
  Product1 : Product
  Switch5 : Switch  Threshold=400  SaturateOnIntegerOverflow=off  InputSameDT=off
  Thermal Conductivity : Lookup_n-D  NumberOfTableDimensions=1  BreakpointsForDimension1=PlntThrCoolCpBpt  Table=PlntThrCoolCond  ExtrapMethod=Clip  UseLastTableValue=on  InternalRulePriority=Speed  RndMeth=Simplest
  Vector Concatenate : Concatenate
  Vector Concatenate1 : Concatenate
  HTC : Outport
  wires:
  LPF with IC1/1(y) -> HTC/1  "HTCest"
  FluidTemp/1 -> Prandtl Number/1, [CoolTemp], Abs Viscosity/1
  [CoolTemp] -> Thermal Conductivity/1
  MassFlow/1 -> Divide/1
  HydDia/1 -> [HydD], Divide/2
  CrossA/1 -> Divide/3
  [HydD] -> Divide2/1
  TubLen/1 -> Divide2/2
  Divide2/1 -> [DoL]
  Abs Viscosity/1 -> Divide/4
  Divide/1 -> Vector Concatenate1/1  "ReD"
  Prandtl Number/1 -> Vector Concatenate1/2
  Vector Concatenate1/1 -> Calculation1/1
  [DoL] -> Math Function/1
  Math Function/1 -> Switch5/2
  Thermal Conductivity/1 -> Divide3/1
  [HydD] -> Divide3/2
  Divide3/1 -> Product1/1
  Gain/1 -> Switch5/1
  Calculation1/1 -> [RePr], Gain/1
  [RePr] -> Vector Concatenate/1
  [DoL] -> Vector Concatenate/2
  Vector Concatenate/1 -> Calculation2/1
  Calculation2/1 -> Switch5/3
  Switch5/1 -> Product1/2  "NuD"
  Product1/1 -> LPF with IC1/1(u)

== system ElectricalThermalSystem/Motor/TwoEMs/EM1/Temperature and Heat Flow ==
  HTC : Inport
  CoolTempIn : Inport  Port=2
  EMTemp : Inport  Port=3
  CoolMflw : Inport  Port=4
  JacArea : Inport  Port=5
  Divide2 : Product  Inputs=*/
  Gain4 : Gain  Gain=0.5
  LPF with IC1 : Subsystem  mask{wc=10, InitCond=EnvAirTemp, dataType=off}
      mask prompts: wc "Cutoff frequency, wc [rad/s]"; InitCond "Initial condition, InitCond [same as u]"; dataType "Enforce same input data type"
      mask TypeOptions wc: Cont LPF IC/wc
      mask TypeOptions InitCond: Initial Condition/Value
      mask TypeOptions dataType: Cont LPF IC/dataType
  Minus3 : Sum
  Minus4 : Sum
  Product1 : Product  Inputs=3
  Product2 : Product
  Selector : Selector  InputPortWidth=PlntEMNum  IndexOptions=Index vector (dialog)  Indices=1  OutputSizes=1
  Specific Heat 2 : Lookup_n-D  NumberOfTableDimensions=1  BreakpointsForDimension1=PlntThrCoolCpBpt  Table=PlntThrCoolCp  ExtrapMethod=Clip  UseLastTableValue=on  InternalRulePriority=Speed  RndMeth=Simplest
  Subtract : Sum  Inputs=+-
  div0protect - abs poly4 : autolibutils/div0protect - abs poly  thresh=.001  aMode=1
  BulkCoolTemp : Outport
  Qem : Outport  Port=2
  CoolTempOut : Outport  Port=3
  wires:
  LPF with IC1/1(y) -> BulkCoolTemp/1, [BulkCoolTemp]
  EMTemp/1 -> Selector/1
  HTC/1 -> Product1/1
  Product2/1 -> div0protect - abs poly4/1
  Minus4/1 -> Gain4/1
  Gain4/1 -> LPF with IC1/1(u)
  Minus3/1 -> Minus4/2, CoolTempOut/1
  Product1/1 -> Divide2/1, Qem/1  "Qem"
  JacArea/1 -> Product1/2
  div0protect - abs poly4/1 -> Divide2/2
  Specific Heat 2/1 -> Product2/2
  [BulkCoolTemp] -> Specific Heat 2/1, Subtract/2
  Subtract/1 -> Product1/3
  Selector/1 -> Subtract/1
  Divide2/1 -> Minus3/2
  CoolMflw/1 -> Product2/1
  CoolTempIn/1 -> Minus4/1, Minus3/1

== system ElectricalThermalSystem/Motor/TwoEMs/EM2/HTC Estimator EM ==
  FluidTemp : Inport
  MassFlow : Inport  Port=2
  CrossA : Inport  Port=3  OutMin=eps
  HydDia : Inport  Port=4
  TubLen : Inport  Port=5
  Abs Viscosity : Lookup_n-D  NumberOfTableDimensions=1  BreakpointsForDimension1=PlntThrCoolCpBpt  Table=PlntThrCoolVisc  ExtrapMethod=Clip  UseLastTableValue=on  InternalRulePriority=Speed  RndMeth=Simplest
  Calculation1 : Fcn  Expr=u(1)^0.8*u(2)^0.33
  Calculation2 : Fcn  Expr=0.036*u(1)*u(2)^0.055
  Divide : Product  Inputs=**//
  Divide2 : Product  Inputs=*/
  Divide3 : Product  Inputs=*/
  Gain : Gain  Gain=0.023
  LPF with IC1 : Subsystem  mask{wc=10, InitCond=10, dataType=off}
      mask prompts: wc "Cutoff frequency, wc [rad/s]"; InitCond "Initial condition, InitCond [same as u]"; dataType "Enforce same input data type"
      mask TypeOptions wc: Cont LPF IC/wc
      mask TypeOptions InitCond: Initial Condition/Value
      mask TypeOptions dataType: Cont LPF IC/dataType
  Math Function : Math  Operator=reciprocal
  Prandtl Number : Lookup_n-D  NumberOfTableDimensions=1  BreakpointsForDimension1=PlntThrCoolCpBpt  Table=PlntThrCoolPrand  ExtrapMethod=Clip  UseLastTableValue=on  InternalRulePriority=Speed  RndMeth=Simplest
  Product1 : Product
  Switch5 : Switch  Threshold=400  SaturateOnIntegerOverflow=off  InputSameDT=off
  Thermal Conductivity : Lookup_n-D  NumberOfTableDimensions=1  BreakpointsForDimension1=PlntThrCoolCpBpt  Table=PlntThrCoolCond  ExtrapMethod=Clip  UseLastTableValue=on  InternalRulePriority=Speed  RndMeth=Simplest
  Vector Concatenate : Concatenate
  Vector Concatenate1 : Concatenate
  HTC : Outport
  wires:
  LPF with IC1/1(y) -> HTC/1  "HTCest"
  FluidTemp/1 -> Prandtl Number/1, [CoolTemp], Abs Viscosity/1
  [CoolTemp] -> Thermal Conductivity/1
  MassFlow/1 -> Divide/1
  HydDia/1 -> [HydD], Divide/2
  CrossA/1 -> Divide/3
  [HydD] -> Divide2/1
  TubLen/1 -> Divide2/2
  Divide2/1 -> [DoL]
  Abs Viscosity/1 -> Divide/4
  Divide/1 -> Vector Concatenate1/1  "ReD"
  Prandtl Number/1 -> Vector Concatenate1/2
  Vector Concatenate1/1 -> Calculation1/1
  [DoL] -> Math Function/1
  Math Function/1 -> Switch5/2
  Thermal Conductivity/1 -> Divide3/1
  [HydD] -> Divide3/2
  Divide3/1 -> Product1/1
  Gain/1 -> Switch5/1
  Calculation1/1 -> [RePr], Gain/1
  [RePr] -> Vector Concatenate/1
  [DoL] -> Vector Concatenate/2
  Vector Concatenate/1 -> Calculation2/1
  Calculation2/1 -> Switch5/3
  Switch5/1 -> Product1/2  "NuD"
  Product1/1 -> LPF with IC1/1(u)

== system ElectricalThermalSystem/Motor/TwoEMs/EM2/Temperature and Heat Flow ==
  HTC : Inport
  CoolTempIn : Inport  Port=2
  EMTemp : Inport  Port=3
  CoolMflw : Inport  Port=4
  JacArea : Inport  Port=5
  Divide2 : Product  Inputs=*/
  Gain4 : Gain  Gain=0.5
  LPF with IC1 : Subsystem  mask{wc=10, InitCond=EnvAirTemp, dataType=off}
      mask prompts: wc "Cutoff frequency, wc [rad/s]"; InitCond "Initial condition, InitCond [same as u]"; dataType "Enforce same input data type"
      mask TypeOptions wc: Cont LPF IC/wc
      mask TypeOptions InitCond: Initial Condition/Value
      mask TypeOptions dataType: Cont LPF IC/dataType
  Minus3 : Sum
  Minus4 : Sum
  Product1 : Product  Inputs=3
  Product2 : Product
  Selector : Selector  InputPortWidth=PlntEMNum  IndexOptions=Index vector (dialog)  Indices=2  OutputSizes=1
  Specific Heat 2 : Lookup_n-D  NumberOfTableDimensions=1  BreakpointsForDimension1=PlntThrCoolCpBpt  Table=PlntThrCoolCp  ExtrapMethod=Clip  UseLastTableValue=on  InternalRulePriority=Speed  RndMeth=Simplest
  Subtract : Sum  Inputs=+-
  div0protect - abs poly4 : autolibutils/div0protect - abs poly  thresh=.001  aMode=1
  BulkCoolTemp : Outport
  Qem : Outport  Port=2
  CoolTempOut : Outport  Port=3
  wires:
  LPF with IC1/1(y) -> BulkCoolTemp/1, [BulkCoolTemp]
  EMTemp/1 -> Selector/1
  HTC/1 -> Product1/1
  Product2/1 -> div0protect - abs poly4/1
  Minus4/1 -> Gain4/1
  Gain4/1 -> LPF with IC1/1(u)
  Minus3/1 -> Minus4/2, CoolTempOut/1
  Product1/1 -> Divide2/1, Qem/1  "Qem"
  JacArea/1 -> Product1/2
  div0protect - abs poly4/1 -> Divide2/2
  Specific Heat 2/1 -> Product2/2
  [BulkCoolTemp] -> Specific Heat 2/1, Subtract/2
  Subtract/1 -> Product1/3
  Selector/1 -> Subtract/1
  Divide2/1 -> Minus3/2
  CoolMflw/1 -> Product2/1
  CoolTempIn/1 -> Minus4/1, Minus3/1

== system ElectricalThermalSystem/Front Side HXs/Radiator/NTU and Dimensions/HTC Estimator Air/LPF with IC1 ==
  u : Inport
  Cont LPF IC : autolibutils/Cont LPF IC  wc=wc  aMode=1  dataType=off
  Initial Condition : Constant  Value=InitCond  SampleTime=-1
  y : Outport
  wires:
  Cont LPF IC/1 -> y/1
  u/1 -> Cont LPF IC/1
  Initial Condition/1 -> Cont LPF IC/2

== system ElectricalThermalSystem/Front Side HXs/Radiator/NTU and Dimensions/HTC Estimator Coolant/LPF with IC1 ==
  u : Inport
  Cont LPF IC : autolibutils/Cont LPF IC  wc=wc  aMode=1  dataType=off
  Initial Condition : Constant  Value=InitCond  SampleTime=-1
  y : Outport
  wires:
  Cont LPF IC/1 -> y/1
  u/1 -> Cont LPF IC/1
  Initial Condition/1 -> Cont LPF IC/2

== system ElectricalThermalSystem/Motor/FourEMs/EM1/HTC Estimator EM/LPF with IC1 ==
  u : Inport
  Cont LPF IC : autolibutils/Cont LPF IC  wc=wc  aMode=1  dataType=off
  Initial Condition : Constant  Value=InitCond  SampleTime=-1
  y : Outport
  wires:
  Cont LPF IC/1 -> y/1
  u/1 -> Cont LPF IC/1
  Initial Condition/1 -> Cont LPF IC/2

== system ElectricalThermalSystem/Motor/FourEMs/EM1/Temperature and Heat Flow/LPF with IC1 ==
  u : Inport
  Cont LPF IC : autolibutils/Cont LPF IC  wc=wc  aMode=1  dataType=off
  Initial Condition : Constant  Value=InitCond  SampleTime=-1
  y : Outport
  wires:
  Cont LPF IC/1 -> y/1
  u/1 -> Cont LPF IC/1
  Initial Condition/1 -> Cont LPF IC/2

== system ElectricalThermalSystem/Motor/FourEMs/EM2/HTC Estimator EM/LPF with IC1 ==
  u : Inport
  Cont LPF IC : autolibutils/Cont LPF IC  wc=wc  aMode=1  dataType=off
  Initial Condition : Constant  Value=InitCond  SampleTime=-1
  y : Outport
  wires:
  Cont LPF IC/1 -> y/1
  u/1 -> Cont LPF IC/1
  Initial Condition/1 -> Cont LPF IC/2

== system ElectricalThermalSystem/Motor/FourEMs/EM2/Temperature and Heat Flow/LPF with IC1 ==
  u : Inport
  Cont LPF IC : autolibutils/Cont LPF IC  wc=wc  aMode=1  dataType=off
  Initial Condition : Constant  Value=InitCond  SampleTime=-1
  y : Outport
  wires:
  Cont LPF IC/1 -> y/1
  u/1 -> Cont LPF IC/1
  Initial Condition/1 -> Cont LPF IC/2

== system ElectricalThermalSystem/Motor/FourEMs/EM3/HTC Estimator EM/LPF with IC1 ==
  u : Inport
  Cont LPF IC : autolibutils/Cont LPF IC  wc=wc  aMode=1  dataType=off
  Initial Condition : Constant  Value=InitCond  SampleTime=-1
  y : Outport
  wires:
  Cont LPF IC/1 -> y/1
  u/1 -> Cont LPF IC/1
  Initial Condition/1 -> Cont LPF IC/2

== system ElectricalThermalSystem/Motor/FourEMs/EM3/Temperature and Heat Flow/LPF with IC1 ==
  u : Inport
  Cont LPF IC : autolibutils/Cont LPF IC  wc=wc  aMode=1  dataType=off
  Initial Condition : Constant  Value=InitCond  SampleTime=-1
  y : Outport
  wires:
  Cont LPF IC/1 -> y/1
  u/1 -> Cont LPF IC/1
  Initial Condition/1 -> Cont LPF IC/2

== system ElectricalThermalSystem/Motor/FourEMs/EM4/HTC Estimator EM/LPF with IC1 ==
  u : Inport
  Cont LPF IC : autolibutils/Cont LPF IC  wc=wc  aMode=1  dataType=off
  Initial Condition : Constant  Value=InitCond  SampleTime=-1
  y : Outport
  wires:
  Cont LPF IC/1 -> y/1
  u/1 -> Cont LPF IC/1
  Initial Condition/1 -> Cont LPF IC/2

== system ElectricalThermalSystem/Motor/FourEMs/EM4/Temperature and Heat Flow/LPF with IC1 ==
  u : Inport
  Cont LPF IC : autolibutils/Cont LPF IC  wc=wc  aMode=1  dataType=off
  Initial Condition : Constant  Value=InitCond  SampleTime=-1
  y : Outport
  wires:
  Cont LPF IC/1 -> y/1
  u/1 -> Cont LPF IC/1
  Initial Condition/1 -> Cont LPF IC/2

== system ElectricalThermalSystem/Motor/OneEM/EM1/HTC Estimator EM/LPF with IC1 ==
  u : Inport
  Cont LPF IC : autolibutils/Cont LPF IC  wc=wc  aMode=1  dataType=off
  Initial Condition : Constant  Value=InitCond  SampleTime=-1
  y : Outport
  wires:
  Cont LPF IC/1 -> y/1
  u/1 -> Cont LPF IC/1
  Initial Condition/1 -> Cont LPF IC/2

== system ElectricalThermalSystem/Motor/OneEM/EM1/Temperature and Heat Flow/LPF with IC1 ==
  u : Inport
  Cont LPF IC : autolibutils/Cont LPF IC  wc=wc  aMode=1  dataType=off
  Initial Condition : Constant  Value=InitCond  SampleTime=-1
  y : Outport
  wires:
  Cont LPF IC/1 -> y/1
  u/1 -> Cont LPF IC/1
  Initial Condition/1 -> Cont LPF IC/2

== system ElectricalThermalSystem/Motor/ThreeEMs/EM1/HTC Estimator EM/LPF with IC1 ==
  u : Inport
  Cont LPF IC : autolibutils/Cont LPF IC  wc=wc  aMode=1  dataType=off
  Initial Condition : Constant  Value=InitCond  SampleTime=-1
  y : Outport
  wires:
  Cont LPF IC/1 -> y/1
  u/1 -> Cont LPF IC/1
  Initial Condition/1 -> Cont LPF IC/2

== system ElectricalThermalSystem/Motor/ThreeEMs/EM1/Temperature and Heat Flow/LPF with IC1 ==
  u : Inport
  Cont LPF IC : autolibutils/Cont LPF IC  wc=wc  aMode=1  dataType=off
  Initial Condition : Constant  Value=InitCond  SampleTime=-1
  y : Outport
  wires:
  Cont LPF IC/1 -> y/1
  u/1 -> Cont LPF IC/1
  Initial Condition/1 -> Cont LPF IC/2

== system ElectricalThermalSystem/Motor/ThreeEMs/EM2/HTC Estimator EM/LPF with IC1 ==
  u : Inport
  Cont LPF IC : autolibutils/Cont LPF IC  wc=wc  aMode=1  dataType=off
  Initial Condition : Constant  Value=InitCond  SampleTime=-1
  y : Outport
  wires:
  Cont LPF IC/1 -> y/1
  u/1 -> Cont LPF IC/1
  Initial Condition/1 -> Cont LPF IC/2

== system ElectricalThermalSystem/Motor/ThreeEMs/EM2/Temperature and Heat Flow/LPF with IC1 ==
  u : Inport
  Cont LPF IC : autolibutils/Cont LPF IC  wc=wc  aMode=1  dataType=off
  Initial Condition : Constant  Value=InitCond  SampleTime=-1
  y : Outport
  wires:
  Cont LPF IC/1 -> y/1
  u/1 -> Cont LPF IC/1
  Initial Condition/1 -> Cont LPF IC/2

== system ElectricalThermalSystem/Motor/ThreeEMs/EM3/HTC Estimator EM/LPF with IC1 ==
  u : Inport
  Cont LPF IC : autolibutils/Cont LPF IC  wc=wc  aMode=1  dataType=off
  Initial Condition : Constant  Value=InitCond  SampleTime=-1
  y : Outport
  wires:
  Cont LPF IC/1 -> y/1
  u/1 -> Cont LPF IC/1
  Initial Condition/1 -> Cont LPF IC/2

== system ElectricalThermalSystem/Motor/ThreeEMs/EM3/Temperature and Heat Flow/LPF with IC1 ==
  u : Inport
  Cont LPF IC : autolibutils/Cont LPF IC  wc=wc  aMode=1  dataType=off
  Initial Condition : Constant  Value=InitCond  SampleTime=-1
  y : Outport
  wires:
  Cont LPF IC/1 -> y/1
  u/1 -> Cont LPF IC/1
  Initial Condition/1 -> Cont LPF IC/2

== system ElectricalThermalSystem/Motor/TwoEMs/EM1/HTC Estimator EM/LPF with IC1 ==
  u : Inport
  Cont LPF IC : autolibutils/Cont LPF IC  wc=wc  aMode=1  dataType=off
  Initial Condition : Constant  Value=InitCond  SampleTime=-1
  y : Outport
  wires:
  Cont LPF IC/1 -> y/1
  u/1 -> Cont LPF IC/1
  Initial Condition/1 -> Cont LPF IC/2

== system ElectricalThermalSystem/Motor/TwoEMs/EM1/Temperature and Heat Flow/LPF with IC1 ==
  u : Inport
  Cont LPF IC : autolibutils/Cont LPF IC  wc=wc  aMode=1  dataType=off
  Initial Condition : Constant  Value=InitCond  SampleTime=-1
  y : Outport
  wires:
  Cont LPF IC/1 -> y/1
  u/1 -> Cont LPF IC/1
  Initial Condition/1 -> Cont LPF IC/2

== system ElectricalThermalSystem/Motor/TwoEMs/EM2/HTC Estimator EM/LPF with IC1 ==
  u : Inport
  Cont LPF IC : autolibutils/Cont LPF IC  wc=wc  aMode=1  dataType=off
  Initial Condition : Constant  Value=InitCond  SampleTime=-1
  y : Outport
  wires:
  Cont LPF IC/1 -> y/1
  u/1 -> Cont LPF IC/1
  Initial Condition/1 -> Cont LPF IC/2

== system ElectricalThermalSystem/Motor/TwoEMs/EM2/Temperature and Heat Flow/LPF with IC1 ==
  u : Inport
  Cont LPF IC : autolibutils/Cont LPF IC  wc=wc  aMode=1  dataType=off
  Initial Condition : Constant  Value=InitCond  SampleTime=-1
  y : Outport
  wires:
  Cont LPF IC/1 -> y/1
  u/1 -> Cont LPF IC/1
  Initial Condition/1 -> Cont LPF IC/2
